simulink model "androidSerialPWMServoSend_Android"  (R2019a)
settings: Solver=FixedStepAuto  StartTime=0.0  StopTime=10.0  RelTol=1e-3
InitFcn:
  | Ts=0.01
undefined symbols (not defined in the file): androidSerialSendReceive, Data_Input, Motor_1, Motor_2, Motor_3, Motor_4, Packet
libraries: androiduilib x6, androidcommunicationlib x1
settings Model: Creator=The MathWorks, Inc.  LastModifiedBy=Alireza
settings OptimizationCC: EnhancedBackFolding=on  PassReuseOutputArgsThreshold=0  MaxStackSize=64  OptimizeBlockOrder=speed  DifferentSizesBufferReuse=on  OptimizationCustomize=off
settings DebuggingCC: ParameterTunabilityLossMsg=error  SymbolicDimsDataTypeCodeGenerationDiagnostic=none
settings HardwareCC: ProdBitPerPointer=32  ProdBitPerSizeT=32  ProdBitPerPtrDiffT=32  ProdLargestAtomicInteger=Long  ProdLargestAtomicFloat=Double  ProdWordSize=32  ProdHWDeviceType=ARM Compatible->ARM Cortex  UseEmbeddedCoderFeatures=off  UseSimulinkCoderFeatures=off
settings SFSimCC: MATLABDynamicMemAlloc=off
settings RTWCC: SystemTargetFile=ert.tlc  HardwareBoard=Android Device  TLCOptions="-aInlineSetEventsForThisBaseRateFcn=TLC_FALSE -aSuppressMultiTaskScheduler=TLC_FALSE  -aRateBasedStepFcn=0"  TemplateMakefile=ert_default_tmf  GenerateReport=on  RTWVerbose=off  Toolchain=Android SDK/NDK Tools  LaunchReport=on
settings CodeAppCC: ForceParamTrailComments=on  OperatorAnnotations=on
settings ERTTargetCC: ERTCustomFileBanners=off  SupportContinuousTime=on  SupportNonInlinedSFcns=on  RemoveResetFunc=off  ModelStepFunctionPrototypeControlCompliant=off

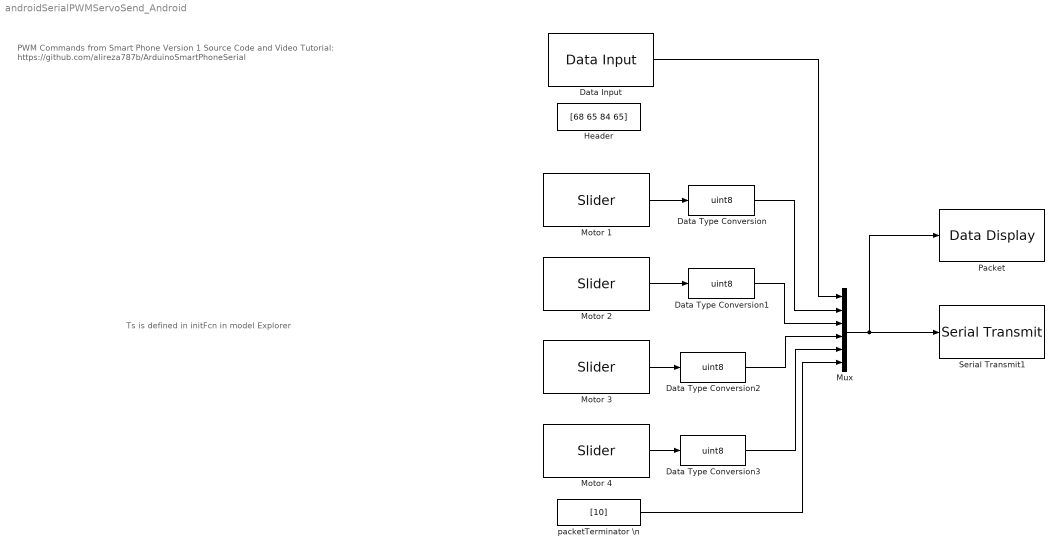
== system androidSerialPWMServoSend_Android ==
  note: PWM Commands from Smart Phone Version 1
      | Source Code and Video Tutorial:
      | https://github.com/alireza787b/ArduinoSmartPhoneSerial
  note: Ts is defined in initFcn in model Explorer
  Data Input : androiduilib/Data Input  isCharVector=on  Value=1.0  CharVector=DATA  OutputDataType=double  maxCharVectorSize=4  DataInputId=androidSerialSendReceive/Data_Input  SampleTime=Ts
      settings: SourceProductBaseCode=ANDROID
  Data Type Conversion{,1..3} (4 alike) : DataTypeConversion  OutDataTypeStr=uint8
  Header : Constant  Value=[68 65 84 65]  OutDataTypeStr=uint8  SampleTime=Ts
  Motor 1 : androiduilib/Slider  Min=0  Value=0  Max=255  Resolution=1  SliderId=androidSerialSendReceive/Motor_1  SampleTime=Ts  BlockPlatform=Android
      settings: SourceProductBaseCode=ANDROID
  Motor 2 : androiduilib/Slider  Min=0  Value=0  Max=255  Resolution=1  SliderId=androidSerialSendReceive/Motor_2  SampleTime=Ts  BlockPlatform=Android
      settings: SourceProductBaseCode=ANDROID
  Motor 3 : androiduilib/Slider  Min=0  Value=0  Max=255  Resolution=1  SliderId=androidSerialSendReceive/Motor_3  SampleTime=Ts  BlockPlatform=Android
      settings: SourceProductBaseCode=ANDROID
  Motor 4 : androiduilib/Slider  Min=0  Value=0  Max=255  Resolution=1  SliderId=androidSerialSendReceive/Motor_4  SampleTime=Ts  BlockPlatform=Android
      settings: SourceProductBaseCode=ANDROID
  Mux : Mux  Inputs=6
  Packet : androiduilib/Data Display  DataDisplayId=androidSerialSendReceive/Packet  Format=Integer  Precision=6  SimulateUsing=Code generation  blockPlatform=Android
      settings: SourceProductBaseCode=ANDROID
  Serial Transmit1 : androidcommunicationlib/Serial Transmit
      settings: SourceProductBaseCode=ANDROID
  packetTerminator \n : Constant  Value=[10]  OutDataTypeStr=uint8
  wires:
  Motor 1/1 -> Data Type Conversion/1
  Motor 4/1 -> Data Type Conversion3/1
  Motor 3/1 -> Data Type Conversion2/1
  Motor 2/1 -> Data Type Conversion1/1
  Data Type Conversion1/1 -> Mux/3
  Data Type Conversion2/1 -> Mux/4
  Data Type Conversion/1 -> Mux/2
  Data Type Conversion3/1 -> Mux/5
  packetTerminator \n/1 -> Mux/6
  Mux/1 -> Packet/1, Serial Transmit1/1
  Data Input/1 -> Mux/1
